simulink model "SMA_spring"  (R2018a)
settings: Solver=ode15s  StartTime=0.0  StopTime=20  RelTol=1e-6  AbsTol=1e-6
settings Model: Creator=Matthias  LastModifiedBy=Matthias

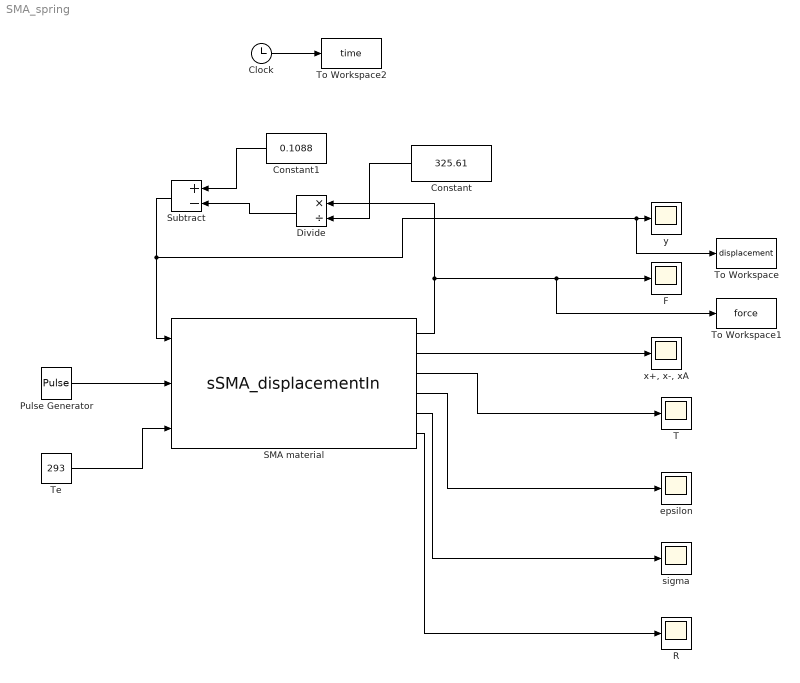
== system SMA_spring ==
  Clock : Clock
  Constant : Constant  Value=325.61
  Constant1 : Constant  Value=0.1088
  Divide : Product  Inputs=*/
  F : Scope
  Pulse Generator : DiscretePulseGenerator  PulseType=Time based  Amplitude=0.4  Period=10  PulseWidth=50
  R : Scope
  SMA material : M-S-Function  FunctionName=sSMA_displacementIn  Parameters=params, initConds
      mask Display:
      | color('black');
      | patch(3*[-1 1 1 -1],1.1*[-1 -1 1 1],[1 1 1]);
      | patch([-1.6 -0.8],[-0.9 0.3],[0 0 0]);
      | patch([-0.8 1.2],[0.3 0.3],[0 0 0]);
      | patch([1.6 0.8],[0.9 -0.3],[0 0 0]);
      | patch([0.8 -1.2],[-0.3 -0.3],[0 0 0]);
      | disp('SMA');
      | 
      | color('blue');
      | port_label('input', 1, 'y [m]','texmode','on');
      | port_label('input', 2, 'J [W]','texmode','on');
      | port_label('input', 3, 'T_E [K]','texmode','on');
      | 
      | color('red');
      | port_label('output', 1, 'F [N]','texmode','on');
      | port_label('output', 2, 'x_+, x_-, x_A [-]','texmode','on');
      | port_label('output', 3, 'T [K]','texmode','on');
      | port_label('output', 4, '\epsilon [-]','texmode','on');
      | port_label('output', 5, '\sigma [Pa]','texmode','on');
      | port_label('output', 6, 'R [\Omega]','texmode','on');
  Subtract : Sum  Inputs=+-
  T : Scope
  Te : Constant  Value=293
  To Workspace : ToWorkspace  VariableName=displacement  SampleTime=-1
  To Workspace1 : ToWorkspace  VariableName=force  SampleTime=-1
  To Workspace2 : ToWorkspace  VariableName=time  SampleTime=-1
  epsilon : Scope
  sigma : Scope
  "x+, x-, xA" : Scope
  y : Scope
  wires:
  SMA material/5 -> sigma/1
  Clock/1 -> To Workspace2/1
  SMA material/4 -> epsilon/1
  SMA material/6 -> R/1
  SMA material/3 -> T/1
  Te/1 -> SMA material/3
  SMA material/1 -> Divide/1, To Workspace1/1, F/1
  SMA material/2 -> "x+, x-, xA"/1
  Pulse Generator/1 -> SMA material/2
  Constant1/1 -> Subtract/1
  Constant/1 -> Divide/2
  Divide/1 -> Subtract/2
  Subtract/1 -> To Workspace/1, y/1, SMA material/1
